simulink model "smartCart5_1work"  (R2016a)
settings: Solver=FixedStepDiscrete  StartTime=0.0  StopTime=inf  FixedStep=1  RelTol=1e-3
libraries: simulink x213, hdlsllib x84
(part 1 of 4)
settings Model: Creator=Admin  LastModifiedBy=4230
settings OptimizationCC: BlockReduction=off  ConditionallyExecuteInputs=off  DefaultParameterBehavior=Inlined
settings DebuggingCC: AlgebraicLoopMsg=error
settings HardwareCC: ProdBitPerPointer=32  ProdLargestAtomicFloat=None  ProdIntDivRoundTo=Undefined  ProdEndianess=Unspecified  ProdWordSize=32  ProdHWDeviceType=ASIC/FPGA->ASIC/FPGA  ProdEqTarget=off

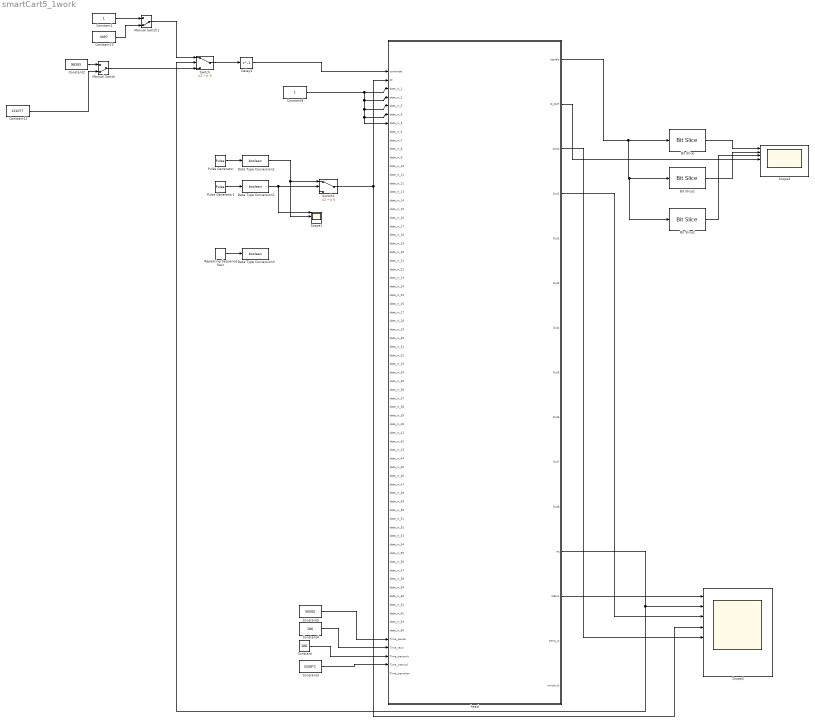
== system smartCart5_1work ==
  Bit Slice : hdlsllib/HDL Operations/Bit Slice  lidx=0  ridx=0
  Bit Slice1 : hdlsllib/HDL Operations/Bit Slice  lidx=1  ridx=1
  Bit Slice2 : hdlsllib/HDL Operations/Bit Slice  lidx=2  ridx=2
  Constant : Constant  Value=186  OutDataTypeStr=uint32  SampleTime=-1
  Constant1 : Constant  OutDataTypeStr=uint32  SampleTime=-1
  Constant12 : Constant  Value=131077  OutDataTypeStr=uint32  SampleTime=-1
  Constant13 : Constant  Value=4097  OutDataTypeStr=uint32  SampleTime=-1
  Constant2 : Constant  Value=98305  OutDataTypeStr=uint32  SampleTime=-1
  Constant3 : Constant  Value=5208*2  OutDataTypeStr=uint32  SampleTime=-1
  Constant4 : Constant  Value=186  OutDataTypeStr=uint32  SampleTime=-1
  Constant5 : Constant  Value=50000  OutDataTypeStr=uint32  SampleTime=-1
  Constant9 : Constant  OutDataTypeStr=uint32  SampleTime=-1
  Data Type Conversion1 : DataTypeConversion  OutDataTypeStr=boolean
  Data Type Conversion2 : DataTypeConversion  OutDataTypeStr=boolean
  Data Type Conversion3 : DataTypeConversion  OutDataTypeStr=boolean
  Delay1 : Delay  DelayLength=1  InitialCondition=0
  Manual Switch : ManualSwitch  CurrentSetting=0
  Manual Switch1 : ManualSwitch  CurrentSetting=0
  Pulse Generator : DiscretePulseGenerator  Period=4  PulseWidth=2
  Pulse Generator1 : DiscretePulseGenerator  Period=500000  PulseWidth=2000
  Repeating Sequence Stair : simulink/Sources/Repeating Sequence Stair  OutValues="[0 0 0 0 1 0 0 0 0 0 0 0 0 0 0 0 0 0 0 0 0 0 0 0 0 0 0 0 0 0 0 0 0 0 0 0 0 0 0 0 0 0 0 0 0 0 0 0  ].'"  tsamp=-1  OutMin=[]  OutMax=[]  OutDataTypeStr=double  OutputDataTypeScalingMode=double  OutDataType=fixdt(0,8)  ConRadixGroup=Best Precision: Vector-wise  OutScaling=2^-12
  Scope1 : Scope  NumInputPorts=4
  Scope2 : Scope  NumInputPorts=8
  Scope3 : Scope  NumInputPorts=8
  Switch : Switch  Criteria=u2 ~= 0
  Switch1 : Switch  Criteria=u2 ~= 0
  head : Subsystem  TreatAsAtomicUnit=on
  wires:
  Switch/1 -> Delay1/1
  Constant2/1 -> Manual Switch/1
  Manual Switch/1 -> Switch/3
  Constant12/1 -> Manual Switch/2
  Constant1/1 -> Manual Switch1/1
  Manual Switch1/1 -> Switch/1
  Constant13/1 -> Manual Switch1/2
  Delay1/1 -> head/1(comanda)
  head/12(irq) -> Scope2/2, Switch/2
  Constant5/1 -> head/67(Time_pause)
  Constant4/1 -> head/68(Time_reciv)
  Constant/1 -> head/69(Time_transmit)
  Constant3/1 -> head/70(Time_interval)
  Constant9/1 -> head/7(data_in_5), head/6(data_in_4), head/5(data_in_3), head/4(data_in_2), head/3(data_in_1)
  Pulse Generator1/1 -> Data Type Conversion1/1
  Data Type Conversion1/1 -> Scope1/1, Switch1/2
  Pulse Generator/1 -> Data Type Conversion2/1
  Data Type Conversion2/1 -> Scope1/2, Switch1/1
  head/13(status) -> Scope2/1
  head/3(strob) -> Scope2/5
  head/4(Out1) -> Scope2/3
  Repeating Sequence Stair/1 -> Data Type Conversion3/1
  Switch1/1 -> Scope2/4, head/2(IO)
  head/1(signals) -> Bit Slice2/1, Bit Slice1/1, Bit Slice/1
  Bit Slice/1 -> Scope3/1
  Bit Slice1/1 -> Scope3/2
  Bit Slice2/1 -> Scope3/3
  head/2(I0_OUT) -> Scope3/4

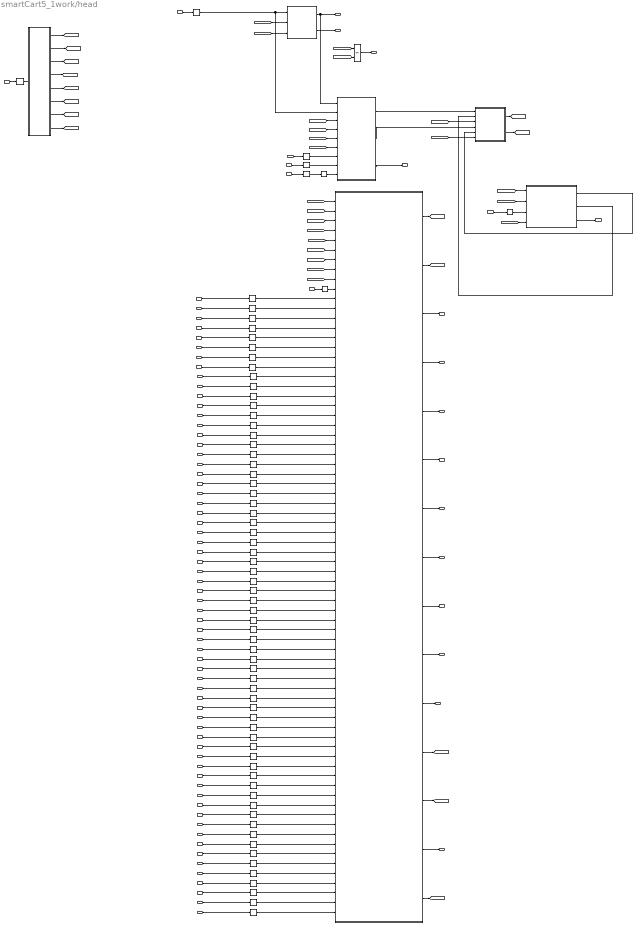
== system smartCart5_1work/head ==
  note: Переключатель адрес 4
  note: Приёмник адрес (1)
      | 1-2 бит   тип сообщения  если  1 то соостояние счётчика  2 считыные байт байты
      | 3-11 бит значение сяётчика адреса
      | 12-20 бит считанный байт
  comanda : Inport  OutDataTypeStr=uint32
  IO : Inport  Port=2  OutDataTypeStr=boolean
  data_in_1 : Inport  Port=3  OutDataTypeStr=uint32
  data_in_2 : Inport  Port=4  OutDataTypeStr=uint32
  data_in_3 : Inport  Port=5  OutDataTypeStr=uint32
  data_in_4 : Inport  Port=6  OutDataTypeStr=uint32
  data_in_5 : Inport  Port=7  OutDataTypeStr=uint32
  data_in_6 : Inport  Port=8  OutDataTypeStr=uint32
  data_in_7 : Inport  Port=9  OutDataTypeStr=uint32
  data_in_8 : Inport  Port=10  OutDataTypeStr=uint32
  data_in_9 : Inport  Port=11  OutDataTypeStr=uint32
  data_in_10 : Inport  Port=12  OutDataTypeStr=uint32
  data_in_11 : Inport  Port=13  OutDataTypeStr=uint32
  data_in_12 : Inport  Port=14  OutDataTypeStr=uint32
  data_in_13 : Inport  Port=15  OutDataTypeStr=uint32
  data_in_14 : Inport  Port=16  OutDataTypeStr=uint32
  data_in_15 : Inport  Port=17  OutDataTypeStr=uint32
  data_in_16 : Inport  Port=18  OutDataTypeStr=uint32
  data_in_17 : Inport  Port=19  OutDataTypeStr=uint32
  data_in_18 : Inport  Port=20  OutDataTypeStr=uint32
  data_in_19 : Inport  Port=21  OutDataTypeStr=uint32
  data_in_20 : Inport  Port=22  OutDataTypeStr=uint32
  data_in_21 : Inport  Port=23  OutDataTypeStr=uint32
  data_in_22 : Inport  Port=24  OutDataTypeStr=uint32
  data_in_23 : Inport  Port=25  OutDataTypeStr=uint32
  data_in_24 : Inport  Port=26  OutDataTypeStr=uint32
  data_in_25 : Inport  Port=27  OutDataTypeStr=uint32
  data_in_26 : Inport  Port=28  OutDataTypeStr=uint32
  data_in_27 : Inport  Port=29  OutDataTypeStr=uint32
  data_in_28 : Inport  Port=30  OutDataTypeStr=uint32
  data_in_29 : Inport  Port=31  OutDataTypeStr=uint32
  data_in_30 : Inport  Port=32  OutDataTypeStr=uint32
  data_in_31 : Inport  Port=33  OutDataTypeStr=uint32
  data_in_32 : Inport  Port=34  OutDataTypeStr=uint32
  data_in_33 : Inport  Port=35  OutDataTypeStr=uint32
  data_in_34 : Inport  Port=36  OutDataTypeStr=uint32
  data_in_35 : Inport  Port=37  OutDataTypeStr=uint32
  data_in_36 : Inport  Port=38  OutDataTypeStr=uint32
  data_in_37 : Inport  Port=39  OutDataTypeStr=uint32
  data_in_38 : Inport  Port=40  OutDataTypeStr=uint32
  data_in_39 : Inport  Port=41  OutDataTypeStr=uint32
  data_in_40 : Inport  Port=42  OutDataTypeStr=uint32
  data_in_41 : Inport  Port=43  OutDataTypeStr=uint32
  data_in_42 : Inport  Port=44  OutDataTypeStr=uint32
  data_in_43 : Inport  Port=45  OutDataTypeStr=uint32
  data_in_44 : Inport  Port=46  OutDataTypeStr=uint32
  data_in_45 : Inport  Port=47  OutDataTypeStr=uint32
  data_in_46 : Inport  Port=48  OutDataTypeStr=uint32
  data_in_47 : Inport  Port=49  OutDataTypeStr=uint32
  data_in_48 : Inport  Port=50  OutDataTypeStr=uint32
  data_in_49 : Inport  Port=51  OutDataTypeStr=uint32
  data_in_50 : Inport  Port=52  OutDataTypeStr=uint32
  data_in_51 : Inport  Port=53  OutDataTypeStr=uint32
  data_in_52 : Inport  Port=54  OutDataTypeStr=uint32
  data_in_53 : Inport  Port=55  OutDataTypeStr=uint32
  data_in_54 : Inport  Port=56  OutDataTypeStr=uint32
  data_in_55 : Inport  Port=57  OutDataTypeStr=uint32
  data_in_56 : Inport  Port=58  OutDataTypeStr=uint32
  data_in_57 : Inport  Port=59  OutDataTypeStr=uint32
  data_in_58 : Inport  Port=60  OutDataTypeStr=uint32
  data_in_59 : Inport  Port=61  OutDataTypeStr=uint32
  data_in_60 : Inport  Port=62  OutDataTypeStr=uint32
  data_in_61 : Inport  Port=63  OutDataTypeStr=uint32
  data_in_62 : Inport  Port=64  OutDataTypeStr=uint32
  data_in_63 : Inport  Port=65  OutDataTypeStr=uint32
  data_in_64 : Inport  Port=66  OutDataTypeStr=uint32
  Time_pause : Inport  Port=67  OutDataTypeStr=uint32
  Time_reciv : Inport  Port=68  OutDataTypeStr=uint32
  Time_transmit : Inport  Port=69  OutDataTypeStr=uint32
  Time_interval : Inport  Port=70  OutDataTypeStr=uint32
  Time_transition : Inport  Port=71  OutDataTypeStr=uint32
  DEMUX : Subsystem  TreatAsAtomicUnit=on
  Delay{,1..71} (72 alike) : Delay  DelayLength=1  InitialCondition=0
  Interface : Subsystem  TreatAsAtomicUnit=on
  Logical Operator : Logic  Operator=OR  AllPortsSameDT=off  OutDataTypeStr=boolean
  MUX : Subsystem  TreatAsAtomicUnit=on
  Manager : Subsystem  TreatAsAtomicUnit=on
  Reciver : Subsystem  TreatAsAtomicUnit=on
  Transmit : Subsystem  TreatAsAtomicUnit=on
  signals : Outport  OutDataTypeStr=fixdt(1,3,0)
  I0_OUT : Outport  Port=2  OutDataTypeStr=boolean
  strob : Outport  Port=3  OutDataTypeStr=boolean
  Out1 : Outport  Port=4  OutDataTypeStr=uint8
  Out2 : Outport  Port=5  OutDataTypeStr=uint8
  Out3 : Outport  Port=6  OutDataTypeStr=uint8
  Out4 : Outport  Port=7  OutDataTypeStr=uint8
  Out5 : Outport  Port=8  OutDataTypeStr=uint8
  Out6 : Outport  Port=9  OutDataTypeStr=uint8
  Out7 : Outport  Port=10  OutDataTypeStr=uint8
  Out8 : Outport  Port=11  OutDataTypeStr=uint8
  irq : Outport  Port=12  OutDataTypeStr=boolean
  status : Outport  Port=13  OutDataTypeStr=uint32
  trans_io : Outport  Port=14  OutDataTypeStr=boolean
  switch_io : Outport  Port=15  OutDataTypeStr=boolean
  wires:
  Interface/1(signals2) -> Reciver/1(RST), signals/1
  Interface/2(Out3) -> I0_OUT/1
  Reciver/3(Strob) -> strob/1
  DEMUX/3(RD_WR) -> [rd_wr]
  Reciver/1(AddrOUT) -> MUX/1(ADR1)
  Reciver/2(STATUS) -> MUX/4(Data1)
  comanda/1 -> Delay/1
  Delay/1 -> DEMUX/1(COMMANDA)
  data_in_1/1 -> Delay2/1
  data_in_2/1 -> Delay3/1
  data_in_3/1 -> Delay4/1
  data_in_4/1 -> Delay5/1
  data_in_5/1 -> Delay6/1
  data_in_6/1 -> Delay7/1
  data_in_7/1 -> Delay8/1
  data_in_8/1 -> Delay9/1
  Transmit/1(DataOUT) -> MUX/5(Data2)
  Transmit/2(addrOUT) -> MUX/2(ADR2)
  IO/1 -> Delay1/1
  Delay1/1 -> Reciver/2(IO), Interface/1(IO)
  Delay10/1 -> Reciver/7(TimOUT)
  Delay11/1 -> Reciver/8(time_transmite)
  Time_transmit/1 -> Delay11/1
  Delay12/1 -> Transmit/3(time_recive)
  Time_reciv/1 -> Delay12/1
  Transmit/3(IO) -> trans_io/1
  Logical Operator/1 -> switch_io/1
  [rd_switch] -> Logical Operator/2
  Delay2/1 -> Manager/11(data_in_0)
  Delay3/1 -> Manager/12(data_in_1)
  Delay4/1 -> Manager/13(data_in_2)
  Delay5/1 -> Manager/14(data_in_3)
  Delay6/1 -> Manager/15(data_in_4)
  Delay7/1 -> Manager/16(data_in_5)
  Delay8/1 -> Manager/17(data_in_6)
  Delay9/1 -> Manager/18(data_in_7)
  data_in_9/1 -> Delay14/1
  data_in_10/1 -> Delay15/1
  data_in_11/1 -> Delay16/1
  data_in_12/1 -> Delay17/1
  data_in_13/1 -> Delay18/1
  data_in_14/1 -> Delay19/1
  data_in_15/1 -> Delay20/1
  data_in_16/1 -> Delay21/1
  Delay14/1 -> Manager/19(data_in_8)
  Delay15/1 -> Manager/20(data_in_9)
  Delay16/1 -> Manager/21(data_in_10)
  Delay17/1 -> Manager/22(data_in_11)
  Delay18/1 -> Manager/23(data_in_12)
  Delay19/1 -> Manager/24(data_in_13)
  Delay20/1 -> Manager/25(data_in_14)
  Delay21/1 -> Manager/26(data_in_15)
  data_in_17/1 -> Delay22/1
  data_in_18/1 -> Delay23/1
  data_in_19/1 -> Delay24/1
  data_in_20/1 -> Delay25/1
  data_in_21/1 -> Delay26/1
  data_in_22/1 -> Delay27/1
  data_in_23/1 -> Delay28/1
  data_in_24/1 -> Delay29/1
  Delay22/1 -> Manager/27(data_in_16)
  Delay23/1 -> Manager/28(data_in_17)
  Delay24/1 -> Manager/29(data_in_18)
  Delay25/1 -> Manager/30(data_in_19)
  Delay26/1 -> Manager/31(data_in_20)
  Delay27/1 -> Manager/32(data_in_21)
  Delay28/1 -> Manager/33(data_in_22)
  Delay29/1 -> Manager/34(data_in_23)
  data_in_25/1 -> Delay30/1
  data_in_26/1 -> Delay31/1
  data_in_27/1 -> Delay32/1
  data_in_28/1 -> Delay33/1
  data_in_29/1 -> Delay34/1
  data_in_30/1 -> Delay35/1
  data_in_31/1 -> Delay36/1
  data_in_32/1 -> Delay37/1
  Delay30/1 -> Manager/35(data_in_24)
  Delay31/1 -> Manager/36(data_in_25)
  Delay32/1 -> Manager/37(data_in_26)
  Delay33/1 -> Manager/38(data_in_27)
  Delay34/1 -> Manager/39(data_in_28)
  Delay35/1 -> Manager/40(data_in_29)
  Delay36/1 -> Manager/41(data_in_30)
  Delay37/1 -> Manager/42(data_in_31)
  data_in_33/1 -> Delay38/1
  data_in_34/1 -> Delay39/1
  data_in_35/1 -> Delay40/1
  data_in_36/1 -> Delay41/1
  data_in_37/1 -> Delay42/1
  data_in_38/1 -> Delay43/1
  data_in_39/1 -> Delay44/1
  data_in_40/1 -> Delay45/1
  Delay38/1 -> Manager/43(data_in_32)
  Delay39/1 -> Manager/44(data_in_33)
  Delay40/1 -> Manager/45(data_in_34)
  Delay41/1 -> Manager/46(data_in_35)
  Delay42/1 -> Manager/47(data_in_36)
  Delay43/1 -> Manager/48(data_in_37)
  Delay44/1 -> Manager/49(data_in_38)
  Delay45/1 -> Manager/50(data_in_39)
  data_in_41/1 -> Delay46/1
  data_in_42/1 -> Delay47/1
  data_in_43/1 -> Delay48/1
  data_in_44/1 -> Delay49/1
  data_in_45/1 -> Delay50/1
  data_in_46/1 -> Delay51/1
  data_in_47/1 -> Delay52/1
  data_in_48/1 -> Delay53/1
  Delay46/1 -> Manager/51(data_in_40)
  Delay47/1 -> Manager/52(data_in_41)
  Delay48/1 -> Manager/53(data_in_42)
  Delay49/1 -> Manager/54(data_in_43)
  Delay50/1 -> Manager/55(data_in_44)
  Delay51/1 -> Manager/56(data_in_45)
  Delay52/1 -> Manager/57(data_in_46)
  Delay53/1 -> Manager/58(data_in_47)
  data_in_49/1 -> Delay54/1
  data_in_50/1 -> Delay55/1
  data_in_51/1 -> Delay56/1
  data_in_52/1 -> Delay57/1
  data_in_53/1 -> Delay58/1
  data_in_54/1 -> Delay59/1
  data_in_55/1 -> Delay60/1
  data_in_56/1 -> Delay61/1
  Delay54/1 -> Manager/59(data_in_48)
  Delay55/1 -> Manager/60(data_in_49)
  Delay56/1 -> Manager/61(data_in_50)
  Delay57/1 -> Manager/62(data_in_51)
  Delay58/1 -> Manager/63(data_in_52)
  Delay59/1 -> Manager/64(data_in_53)
  Delay60/1 -> Manager/65(data_in_54)
  Delay61/1 -> Manager/66(data_in_55)
  data_in_57/1 -> Delay62/1
  data_in_58/1 -> Delay63/1
  data_in_59/1 -> Delay64/1
  data_in_60/1 -> Delay65/1
  data_in_61/1 -> Delay66/1
  data_in_62/1 -> Delay67/1
  data_in_63/1 -> Delay68/1
  data_in_64/1 -> Delay69/1
  Delay62/1 -> Manager/67(data_in_56)
  Delay63/1 -> Manager/68(data_in_57)
  Delay64/1 -> Manager/69(data_in_58)
  Delay65/1 -> Manager/70(data_in_59)
  Delay66/1 -> Manager/71(data_in_60)
  Delay67/1 -> Manager/72(data_in_61)
  Delay68/1 -> Manager/73(data_in_62)
  Delay69/1 -> Manager/74(data_in_63)
  Manager/11(irq) -> irq/1
  Manager/15(rd_switch) -> [rd_switch]
  Manager/14(STATUS) -> status/1
  Delay13/1 -> Manager/10(time_pause)
  Manager/3(Out1) -> Out1/1
  Manager/4(Out2) -> Out2/1
  Manager/5(Out3) -> Out3/1
  Manager/6(Out4) -> Out4/1
  Manager/7(Out5) -> Out5/1
  Manager/8(Out6) -> Out6/1
  Manager/9(Out7) -> Out7/1
  Manager/10(Out8) -> Out8/1
  Manager/13(data_mux) -> [data_mux]
  Manager/12(addr_mux) -> [addr_mux]
  Manager/2(DATA_OUT) -> [data_out]
  Manager/1(addrout) -> [addr_out]
  [data_mux] -> MUX/6(mData3)
  [addr_mux] -> MUX/3(mADR3)
  [addr_out] -> Transmit/1(addrIN)
  [data_out] -> Transmit/2(dataIN)
  [addr_out] -> Reciver/4(adr_IN)
  [data_out] -> Reciver/5(data_in)
  [data_in] -> Manager/2(DataIN)
  [addr_in] -> Manager/1(AdrrIN)
  MUX/2(AdrOut) -> [addr_in]
  MUX/1(DataOut) -> [data_in]
  DEMUX/8(ON_RECIVER) -> [on_reciver]
  [on_reciver] -> Reciver/6(ON_RECIVER)
  DEMUX/7(ON_TRANSMITE) -> [on_transmite]
  [on_transmite] -> Manager/9(ON_TRANSMITE)
  [on_transmite] -> Transmit/4(transmite_on)
  DEMUX/6(Number_write_byte) -> [number_wr_byte]
  [number_wr_byte] -> Manager/8(Number_write_byte)
  [irq_rst] -> Manager/7(RST_IRQ)
  [step] -> Manager/6(STEP)
  [rd_wr] -> Manager/5(RD)
  [start] -> Manager/3(Start)
  [stop] -> Manager/4(Stop)
  DEMUX/5(RST_IRQ) -> [irq_rst]
  DEMUX/4(STEP) -> [step]
  [rd_wr] -> Logical Operator/1
  DEMUX/2(stop) -> [stop]
  [stop] -> Reciver/3(STOP)
  [stop] -> Interface/3(STOP)
  DEMUX/1(start) -> [start]
  [start] -> Interface/2(START)
  Time_pause/1 -> Delay10/1
  Time_interval/1 -> Delay13/1
  Delay70/1 -> Reciver/9(time_transition)
  Delay71/1 -> Delay70/1
  Time_transition/1 -> Delay71/1

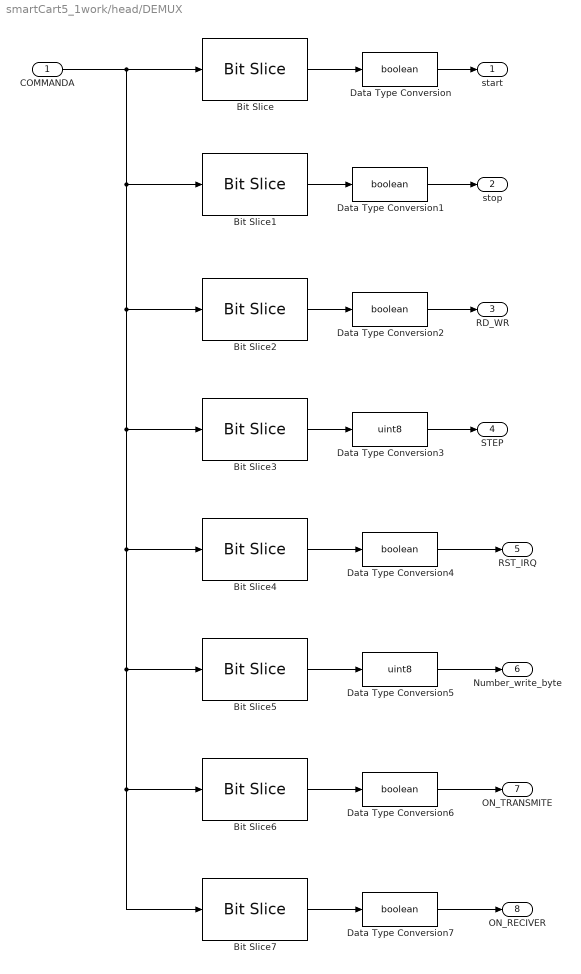
== system smartCart5_1work/head/DEMUX ==
  COMMANDA : Inport  OutDataTypeStr=uint32
  Bit Slice : hdlsllib/HDL Operations/Bit Slice  lidx=0  ridx=0
  Bit Slice1 : hdlsllib/HDL Operations/Bit Slice  lidx=1  ridx=1
  Bit Slice2 : hdlsllib/HDL Operations/Bit Slice  lidx=2  ridx=2
  Bit Slice3 : hdlsllib/HDL Operations/Bit Slice  lidx=11  ridx=3
  Bit Slice4 : hdlsllib/HDL Operations/Bit Slice  lidx=12  ridx=12
  Bit Slice5 : hdlsllib/HDL Operations/Bit Slice  lidx=18  ridx=13
  Bit Slice6 : hdlsllib/HDL Operations/Bit Slice  lidx=19  ridx=19
  Bit Slice7 : hdlsllib/HDL Operations/Bit Slice  lidx=20  ridx=20
  Data Type Conversion{,1..2,4,6..7} (6 alike) : DataTypeConversion  OutDataTypeStr=boolean
  Data Type Conversion3 : DataTypeConversion  OutDataTypeStr=uint8
  Data Type Conversion5 : DataTypeConversion  OutDataTypeStr=uint8
  start : Outport
  stop : Outport  Port=2
  RD_WR : Outport  Port=3
  STEP : Outport  Port=4  OutDataTypeStr=uint8
  RST_IRQ : Outport  Port=5
  Number_write_byte : Outport  Port=6  OutDataTypeStr=uint8
  ON_TRANSMITE : Outport  Port=7  OutDataTypeStr=boolean
  ON_RECIVER : Outport  Port=8  OutDataTypeStr=boolean
  wires:
  Bit Slice/1 -> Data Type Conversion/1
  Data Type Conversion/1 -> start/1
  Bit Slice1/1 -> Data Type Conversion1/1
  Data Type Conversion1/1 -> stop/1
  Bit Slice2/1 -> Data Type Conversion2/1
  Data Type Conversion2/1 -> RD_WR/1
  Bit Slice3/1 -> Data Type Conversion3/1
  Data Type Conversion3/1 -> STEP/1
  Bit Slice4/1 -> Data Type Conversion4/1
  Data Type Conversion4/1 -> RST_IRQ/1
  Bit Slice5/1 -> Data Type Conversion5/1
  Data Type Conversion5/1 -> Number_write_byte/1
  Bit Slice6/1 -> Data Type Conversion6/1
  Data Type Conversion6/1 -> ON_TRANSMITE/1
  Bit Slice7/1 -> Data Type Conversion7/1
  Data Type Conversion7/1 -> ON_RECIVER/1
  COMMANDA/1 -> Bit Slice1/1, Bit Slice5/1, Bit Slice7/1, Bit Slice6/1, Bit Slice4/1, Bit Slice3/1, Bit Slice2/1, Bit Slice/1

== system smartCart5_1work/head/Interface ==
  IO : Inport  OutDataTypeStr=boolean
  START : Inport  Port=2  OutDataTypeStr=boolean
  STOP : Inport  Port=3  OutDataTypeStr=boolean
  ColdStart : Subsystem
  ColdStop2 : Subsystem
  Head2 : Subsystem
  MUX2 : Subsystem
  Swith_signal2 : Subsystem
  signals2 : Outport  OutDataTypeStr=fixdt(1,3,0)  InitialOutput=0
  Out3 : Outport  Port=2  OutDataTypeStr=boolean  InitialOutput=0
  wires:
  IO/1 -> Out3/1, ColdStart/1(Reqest)
  Head2/1(AdrOut) -> Swith_signal2/1(Adr), ColdStart/2(Addr), ColdStop2/1(Addr)
  Head2/2(DataOut) -> Swith_signal2/2(Data), ColdStart/3(Data), ColdStop2/2(Data)
  Swith_signal2/1(OutAddr) -> MUX2/1(ADR)
  ColdStart/2(Signal) -> MUX2/2(DATA_0)
  ColdStop2/2(Signal) -> MUX2/3(DATA_1)
  ColdStart/3(ADR_OUT) -> MUX2/4(ADR_ST)
  ColdStart/1(DataOUT) -> MUX2/5(DAT_ST1)
  ColdStop2/3(ADR_OUT) -> MUX2/6(ADR_STOP)
  ColdStop2/1(DataOUT) -> MUX2/7(DAT_STOP)
  MUX2/2(ADR_OUT) -> Head2/1(ADR_IN)
  MUX2/3(DATA_OUT1) -> Head2/2(DataIN)
  MUX2/1(Signals) -> signals2/1
  START/1 -> Head2/3(START)
  STOP/1 -> Head2/4(STOP)

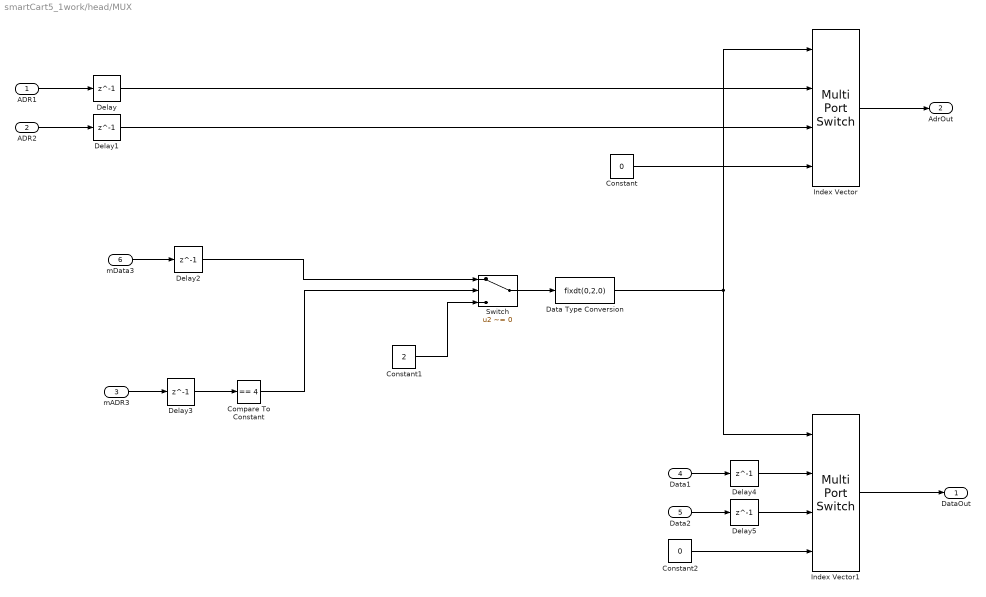
== system smartCart5_1work/head/MUX ==
  ADR1 : Inport  OutDataTypeStr=uint8
  ADR2 : Inport  Port=2  OutDataTypeStr=uint8
  mADR3 : Inport  Port=3  OutDataTypeStr=uint8
  Data1 : Inport  Port=4  OutDataTypeStr=uint32
  Data2 : Inport  Port=5  OutDataTypeStr=uint32
  mData3 : Inport  Port=6  OutDataTypeStr=uint32
  Compare To Constant : simulink/Logic and Bit Operations/Compare To Constant  relop===  const=4  OutDataTypeStr=boolean
  Constant : Constant  Value=0  OutDataTypeStr=uint8
  Constant1 : Constant  Value=2  OutDataTypeStr=uint32
  Constant2 : Constant  Value=0  OutDataTypeStr=uint32
  Data Type Conversion : DataTypeConversion  OutDataTypeStr=fixdt(0,2,0)
  Delay{,1..5} (6 alike) : Delay  DelayLength=1  InitialCondition=0
  Index Vector : MultiPortSwitch  DataPortOrder=Zero-based contiguous  zeroidx=on
  Index Vector1 : MultiPortSwitch  DataPortOrder=Zero-based contiguous  zeroidx=on
  Switch : Switch  Criteria=u2 ~= 0
  DataOut : Outport  OutDataTypeStr=uint32
  AdrOut : Outport  Port=2  OutDataTypeStr=uint8
  wires:
  ADR1/1 -> Delay/1
  ADR2/1 -> Delay1/1
  Constant/1 -> Index Vector/4
  Constant1/1 -> Switch/3
  mData3/1 -> Delay2/1
  Data2/1 -> Delay5/1
  Data1/1 -> Delay4/1
  Constant2/1 -> Index Vector1/4
  Index Vector1/1 -> DataOut/1
  Index Vector/1 -> AdrOut/1
  Switch/1 -> Data Type Conversion/1
  Data Type Conversion/1 -> Index Vector1/1, Index Vector/1
  mADR3/1 -> Delay3/1
  Compare To Constant/1 -> Switch/2
  Delay1/1 -> Index Vector/3
  Delay2/1 -> Switch/1
  Delay3/1 -> Compare To Constant/1
  Delay/1 -> Index Vector/2
  Delay4/1 -> Index Vector1/2
  Delay5/1 -> Index Vector1/3
